simulink model "sampleModel1628"  (R2023a)
settings: Solver=VariableStepAuto  StartTime=0.0  StopTime=10.0  RelTol=1e-3
libraries: hdlsllib x5, simulink x3
settings Model: Creator=user1  LastModifiedBy=user1

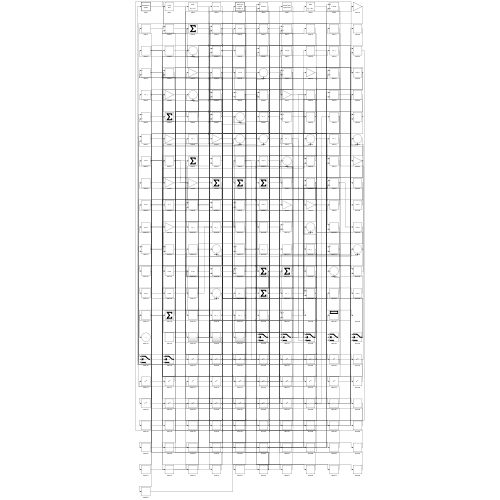
[thumbnail: Simulink's stored preview of the top-level diagram]
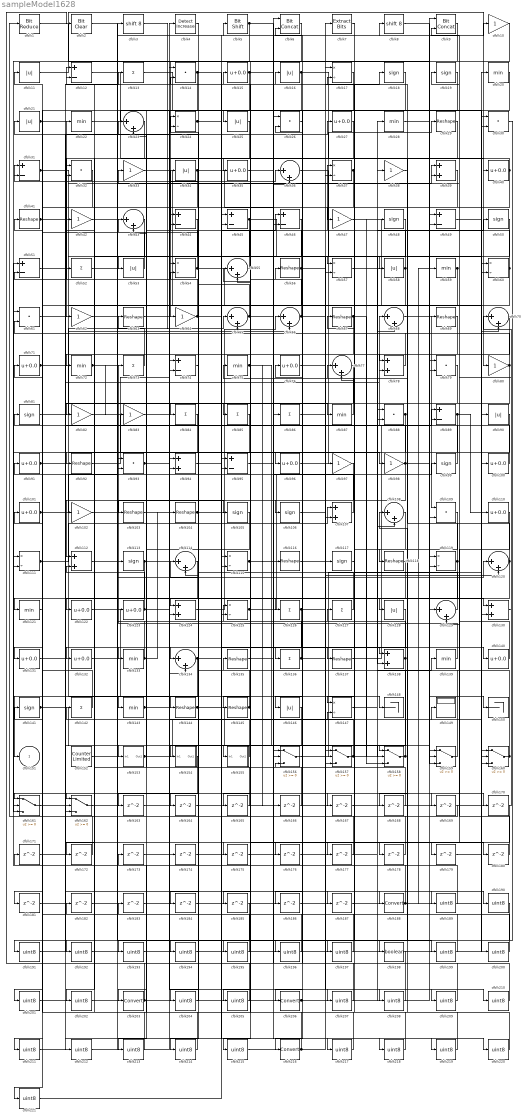
== system sampleModel1628 ==
  cfblk1 : hdlsllib/Logic and Bit Operations/Bit Reduce  mode=AND
  cfblk{10,33,38,42,47,62,64,80,82..83,97..98,102} (13 alike) : Gain
  cfblk{15,27,35,40,71,76,91,96,100..101,110,122..123,131..132,140} (16 alike) : Bias  Bias=0.0  SaturateOnIntegerOverflow=off
  cfblk{29,41,56,63,67,69,92,103..104,116,118,135,137,144..145} (15 alike) : Reshape
  cfblk{18..19,48,50,81,99,105..106,113,117,141} (11 alike) : Signum
  cfblk{39,78,94,107,112,124,130,138} (8 alike) : Sum
  cfblk{23,36,43,55,65..66,68,70,77,108,114,120,129,134} (14 alike) : Sum  Inputs=|++
  cfblk{14,26,30,32,61,79,88,93,109} (9 alike) : DotProduct  OutDataTypeStr=Inherit: Inherit via internal rule
  cfblk{11,16,21,25,34,53,58,90,128,146} (10 alike) : Abs  SaturateOnIntegerOverflow=off
  cfblk{17,24,37,54,57,60,111,115,119,125,147} (11 alike) : Product  Inputs=*/  RndMeth=Zero  SaturateOnIntegerOverflow=on
  cfblk{12,31,44..46,49,51,74,89,95} (10 alike) : Sum  Inputs=+-
  cfblk{20,22,28,59,72,75,87,121,133,139,143} (11 alike) : MinMax
  cfblk{13,52,73,84..86,126..127,136,142} (10 alike) : Sum  Inputs=+
  cfblk148 : Terminator
  cfblk149 : Display
  cfblk150 : Terminator
  cfblk152 : hdlsllib/Sources/Counter Limited  uplimit=7  tsamp=-1
  cfblk153 : Subsystem
      settings: LibrarySourceBlock=|
      | hdlsllib/Ports &
      | Subsystems/Subsystem
  cfblk154 : Subsystem
      settings: LibrarySourceBlock=|
      | hdlsllib/Ports &
      | Subsystems/Subsystem
  cfblk155 : Subsystem
      settings: LibrarySourceBlock=|
      | hdlsllib/Ports &
      | Subsystems/Subsystem
  cfblk{156..162} (7 alike) : Switch  SaturateOnIntegerOverflow=off  InputSameDT=off
  cfblk{163..187} (25 alike) : Delay  SampleTime=1
  cfblk{188,203,206,216} (4 alike) : DataTypeConversion  SaturateOnIntegerOverflow=off  RndMeth=Floor
  cfblk{189..197,199..202,204..205,207..215,217..221} (29 alike) : DataTypeConversion  OutDataTypeStr=uint8  SaturateOnIntegerOverflow=off  RndMeth=Floor
  cfblk198 : DataTypeConversion  OutDataTypeStr=boolean  SaturateOnIntegerOverflow=off  RndMeth=Floor
  cfblk2 : simulink/Logic and Bit Operations/Bit Clear  iBit=0
      settings: LibrarySourceBlock=|
      | hdlsllib/Logic and Bit
      | Operations/Bit Clear
  cfblk3 : ArithShift  BitShiftNumber=8
  cfblk4 : simulink/Logic and Bit Operations/Detect Increase  vinit=0.0  OutDataTypeStr=boolean
      settings: LibrarySourceBlock=|
      | hdlsllib/Logic and Bit
      | Operations/Detect
      | Increase
  cfblk5 : hdlsllib/Logic and Bit Operations/Bit Shift  mode=Shift Left Logical  N=0
  cfblk6 : hdlsllib/Logic and Bit Operations/Bit Concat  numInputs=2
  cfblk7 : simulink/Logic and Bit Operations/Extract Bits  bitsToExtract=Upper half  numBits=8  bitIdxRange=[0 7]  outScalingMode=Preserve fixed-point scaling
      settings: LibrarySourceBlock=|
      | hdlsllib/Logic and Bit
      | Operations/Extract Bits
  cfblk8 : ArithShift  BitShiftNumber=8
  cfblk9 : hdlsllib/Logic and Bit Operations/Bit Concat  numInputs=2
  cfblk151 : Outport  VectorParamsAs1DForOutWhenUnconnected=off
  wires:
  cfblk124/1 -> cfblk66/1
  cfblk5/1 -> cfblk64/1, cfblk158/2, cfblk184/1
  cfblk75/1 -> cfblk158/1, cfblk116/1
  cfblk3/1 -> cfblk65/1
  cfblk64/1 -> cfblk22/1, cfblk218/1
  cfblk100/1 -> cfblk68/1
  cfblk89/1 -> cfblk110/1, cfblk178/1
  cfblk122/1 -> cfblk144/1
  cfblk61/1 -> cfblk66/2
  cfblk51/1 -> cfblk96/1
  cfblk39/1 -> cfblk62/1
  cfblk143/1 -> cfblk5/1, cfblk134/2
  cfblk68/1 -> cfblk109/1
  cfblk125/1 -> cfblk38/1, cfblk55/1
  cfblk133/1 -> cfblk73/1, cfblk104/1
  cfblk111/1 -> cfblk107/1, cfblk78/2
  cfblk11/1 -> cfblk80/1
  cfblk137/1 -> cfblk89/1
  cfblk120/1 -> cfblk75/1, cfblk147/1
  cfblk33/1 -> cfblk115/1
  cfblk17/1 -> cfblk216/1
  cfblk162/1 -> cfblk19/1
  cfblk141/1 -> cfblk153/1(In1), cfblk187/1
  cfblk92/1 -> cfblk4/1
  cfblk27/1 -> cfblk136/1
  cfblk73/1 -> cfblk63/1
  cfblk71/1 -> cfblk148/1, cfblk87/1, cfblk157/2
  cfblk31/1 -> cfblk86/1, cfblk39/2
  cfblk139/1 -> cfblk113/1
  cfblk145/1 -> cfblk91/1, cfblk185/1
  cfblk126/1 -> cfblk155/1(In1), cfblk145/1, cfblk208/1
  cfblk98/1 -> cfblk112/1, cfblk67/1, cfblk150/1
  cfblk22/1 -> cfblk25/1
  cfblk72/1 -> cfblk83/1, cfblk169/1
  cfblk10/1 -> cfblk85/1
  cfblk96/1 -> cfblk29/1
  cfblk81/1 -> cfblk46/1
  cfblk46/1 -> cfblk72/1
  cfblk147/1 -> cfblk50/1
  cfblk76/1 -> cfblk188/1
  cfblk25/1 -> cfblk52/1
  cfblk104/1 -> cfblk69/1, cfblk8/1
  cfblk101/1 -> cfblk93/2, cfblk176/1
  cfblk53/1 -> cfblk11/1
  cfblk134/1 -> cfblk151/1, cfblk65/2
  cfblk54/1 -> cfblk79/1, cfblk31/2
  cfblk153/1(Out1) -> cfblk60/1, cfblk147/2, cfblk149/1
  cfblk119/1 -> cfblk12/1, cfblk133/1
  cfblk23/1 -> cfblk122/1
  cfblk14/1 -> cfblk191/1, cfblk196/1
  cfblk20/1 -> cfblk45/2
  cfblk58/1 -> cfblk16/1, cfblk162/3
  cfblk90/1 -> cfblk132/1
  cfblk1/1 -> cfblk119/2
  cfblk140/1 -> cfblk33/1
  cfblk129/1 -> cfblk77/1
  cfblk135/1 -> cfblk99/1
  cfblk24/1 -> cfblk140/1, cfblk58/1
  cfblk52/1 -> cfblk3/1
  cfblk127/1 -> cfblk43/1
  cfblk74/1 -> cfblk24/1
  cfblk66/1 -> cfblk117/1, cfblk14/2
  cfblk8/1 -> cfblk159/1
  cfblk158/1 -> cfblk21/1, cfblk31/1
  cfblk87/1 -> cfblk15/1
  cfblk42/1 -> cfblk68/2
  cfblk63/1 -> cfblk128/1
  cfblk55/1 -> cfblk34/1
  cfblk57/1 -> cfblk100/1
  cfblk21/1 -> cfblk124/1, cfblk13/1, cfblk177/1
  cfblk44/1 -> cfblk162/1
  cfblk138/1 -> cfblk154/1(In1), cfblk123/1
  cfblk85/1 -> cfblk115/2
  cfblk117/1 -> cfblk77/2
  cfblk80/1 -> cfblk109/2, cfblk61/2, cfblk186/1
  cfblk86/1 -> cfblk7/1
  cfblk59/1 -> cfblk84/1, cfblk121/1
  cfblk12/1 -> cfblk160/2
  cfblk28/1 -> cfblk130/1
  cfblk62/1 -> cfblk105/1
  cfblk78/1 -> cfblk56/1
  cfblk93/1 -> cfblk36/1, cfblk130/2
  cfblk79/1 -> cfblk103/1
  cfblk116/1 -> cfblk18/1
  cfblk156/1 -> cfblk20/1
  cfblk18/1 -> cfblk106/1
  cfblk50/1 -> cfblk138/1
  cfblk37/1 -> cfblk156/2, cfblk202/1
  cfblk67/1 -> cfblk146/1, cfblk158/3
  cfblk159/1 -> cfblk81/1
  cfblk41/1 -> cfblk108/2, cfblk180/1
  cfblk69/1 -> cfblk92/1
  cfblk152/1 -> cfblk120/1
  cfblk16/1 -> cfblk40/1, cfblk53/1
  cfblk15/1 -> cfblk57/1, cfblk43/2
  cfblk128/1 -> cfblk162/2
  cfblk114/1 -> cfblk203/1
  cfblk130/1 -> cfblk70/1
  cfblk144/1 -> cfblk54/2, cfblk159/3
  cfblk84/1 -> cfblk161/1
  cfblk82/1 -> cfblk138/2
  cfblk109/1 -> cfblk118/1
  cfblk91/1 -> cfblk89/2, cfblk217/1
  cfblk99/1 -> cfblk32/1
  cfblk7/1 -> cfblk137/1
  cfblk157/1 -> cfblk125/1, cfblk139/1, cfblk127/1, cfblk48/1
  cfblk45/1 -> cfblk57/2, cfblk74/2, cfblk165/1
  cfblk115/1 -> cfblk36/2, cfblk166/1
  cfblk136/1 -> cfblk120/2, cfblk55/2
  cfblk48/1 -> cfblk143/1
  cfblk13/1 -> cfblk70/2
  cfblk131/1 -> cfblk27/1
  cfblk32/1 -> cfblk131/1
  cfblk113/1 -> cfblk14/1, cfblk161/2
  cfblk107/1 -> cfblk23/1
  cfblk43/1 -> cfblk82/1
  cfblk60/1 -> cfblk37/1, cfblk163/1
  cfblk65/1 -> cfblk39/1, cfblk44/2
  cfblk36/1 -> cfblk90/1
  cfblk88/1 -> cfblk125/2, cfblk161/3
  cfblk34/1 -> cfblk46/2, cfblk134/1, cfblk44/1
  cfblk26/1 -> cfblk206/1
  cfblk123/1 -> cfblk112/2, cfblk207/1
  cfblk155/1(Out1) -> cfblk142/1
  cfblk160/1 -> cfblk51/2, cfblk129/2
  cfblk19/1 -> cfblk124/2
  cfblk47/1 -> cfblk129/1
  cfblk56/1 -> cfblk98/1, cfblk32/2, cfblk126/1, cfblk201/1
  cfblk40/1 -> cfblk78/1, cfblk35/1, cfblk47/1
  cfblk9/1 -> cfblk111/2
  cfblk112/1 -> cfblk10/1
  cfblk142/1 -> cfblk71/1
  cfblk163/1 -> cfblk79/2
  cfblk118/1 -> cfblk164/1
  cfblk164/1 -> cfblk156/1
  cfblk165/1 -> cfblk23/2
  cfblk166/1 -> cfblk12/2
  cfblk132/1 -> cfblk167/1
  cfblk167/1 -> cfblk119/1
  cfblk38/1 -> cfblk168/1
  cfblk168/1 -> cfblk45/1
  cfblk169/1 -> cfblk1/1
  cfblk83/1 -> cfblk170/1
  cfblk77/1 -> cfblk172/1
  cfblk172/1 -> cfblk51/1
  cfblk173/1 -> cfblk24/2
  cfblk174/1 -> cfblk88/2
  cfblk161/1 -> cfblk175/1
  cfblk175/1 -> cfblk107/2
  cfblk176/1 -> cfblk37/2
  cfblk177/1 -> cfblk74/1
  cfblk178/1 -> cfblk111/1
  cfblk110/1 -> cfblk179/1
  cfblk179/1 -> cfblk160/1
  cfblk180/1 -> cfblk9/2
  cfblk121/1 -> cfblk181/1
  cfblk181/1 -> cfblk54/1
  cfblk182/1 -> cfblk157/1
  cfblk183/1 -> cfblk60/2
  cfblk184/1 -> cfblk157/3
  cfblk186/1 -> cfblk156/3
  cfblk187/1 -> cfblk160/3
  cfblk188/1 -> cfblk61/1, cfblk59/1
  cfblk106/1 -> cfblk189/1
  cfblk189/1 -> cfblk76/1
  cfblk102/1 -> cfblk190/1
  cfblk191/1 -> cfblk102/1
  cfblk30/1 -> cfblk192/1
  cfblk192/1 -> cfblk174/1
  cfblk190/1 -> cfblk193/1
  cfblk193/1 -> cfblk30/1
  cfblk4/1 -> cfblk194/1
  cfblk194/1 -> cfblk30/2
  cfblk6/1 -> cfblk195/1
  cfblk195/1 -> cfblk173/1
  cfblk196/1 -> cfblk6/1
  cfblk108/1 -> cfblk197/1
  cfblk197/1 -> cfblk6/2
  cfblk29/1 -> cfblk198/1
  cfblk198/1 -> cfblk2/1
  cfblk2/1 -> cfblk199/1
  cfblk199/1 -> cfblk9/1
  cfblk49/1 -> cfblk200/1
  cfblk200/1 -> cfblk41/1
  cfblk201/1 -> cfblk49/1
  cfblk202/1 -> cfblk49/2
  cfblk203/1 -> cfblk42/1, cfblk88/1
  cfblk70/1 -> cfblk204/1
  cfblk204/1 -> cfblk114/1
  cfblk170/1 -> cfblk205/1
  cfblk205/1 -> cfblk114/2
  cfblk206/1 -> cfblk159/2, cfblk28/1
  cfblk207/1 -> cfblk26/1
  cfblk208/1 -> cfblk26/2
  cfblk94/1 -> cfblk209/1
  cfblk209/1 -> cfblk141/1
  cfblk103/1 -> cfblk210/1
  cfblk210/1 -> cfblk94/1
  cfblk185/1 -> cfblk211/1
  cfblk211/1 -> cfblk94/2
  cfblk171/1 -> cfblk212/1
  cfblk212/1 -> cfblk93/1
  cfblk105/1 -> cfblk213/1
  cfblk213/1 -> cfblk171/1
  cfblk97/1 -> cfblk214/1
  cfblk214/1 -> cfblk101/1
  cfblk146/1 -> cfblk215/1
  cfblk215/1 -> cfblk97/1
  cfblk216/1 -> cfblk183/1, cfblk182/1, cfblk135/1
  cfblk217/1 -> cfblk17/1
  cfblk218/1 -> cfblk17/2
  cfblk95/1 -> cfblk219/1
  cfblk219/1 -> cfblk108/1
  cfblk35/1 -> cfblk220/1
  cfblk220/1 -> cfblk95/1
  cfblk154/1(Out1) -> cfblk221/1
  cfblk221/1 -> cfblk95/2

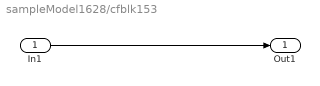
== system sampleModel1628/cfblk153 ==
  In1 : Inport
  Out1 : Outport
  wires:
  In1/1 -> Out1/1

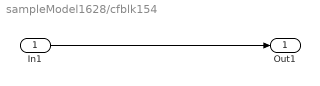
== system sampleModel1628/cfblk154 ==
  In1 : Inport
  Out1 : Outport
  wires:
  In1/1 -> Out1/1

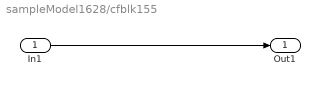
== system sampleModel1628/cfblk155 ==
  In1 : Inport
  Out1 : Outport
  wires:
  In1/1 -> Out1/1
